simulink model "HPGR_2"  (Simulink 7.5)
settings: Solver=ode45  StartTime=0.0  StopTime=10.0  RelTol=1e-3
values from neighbouring files (symbols this model uses):
  n = 13    [CHANCADO_HPGR.m]    (also in Eficiencia_harnero_flujos.m; Granulometria10a.m; HARNERO_bajo_Tamano.m; Prechancado.m)
  X = [37.649701194 26.5631323454 18.9314553059 13.3865604245 9.46572765296 6.69328021227 3.95979797464 1.67332005307 0.707106781187 0.39686269666 0.25099800796 0.158113883008 ... (13 elements, 1x13)]    [matlab.mat]
  Xc = (s0 + D*(1-cos(alfaIP*pi/180)))*1000    [Capacidad_tratamiento_consumo_energia_especifica.m]    (also in Prechancado.m = 27.6127; programacion.m = x(1))
undefined symbols (not defined in the file or in its folder): alfa, faHPGR
settings Model: Creator=Lucho  LastModifiedBy=Lucho

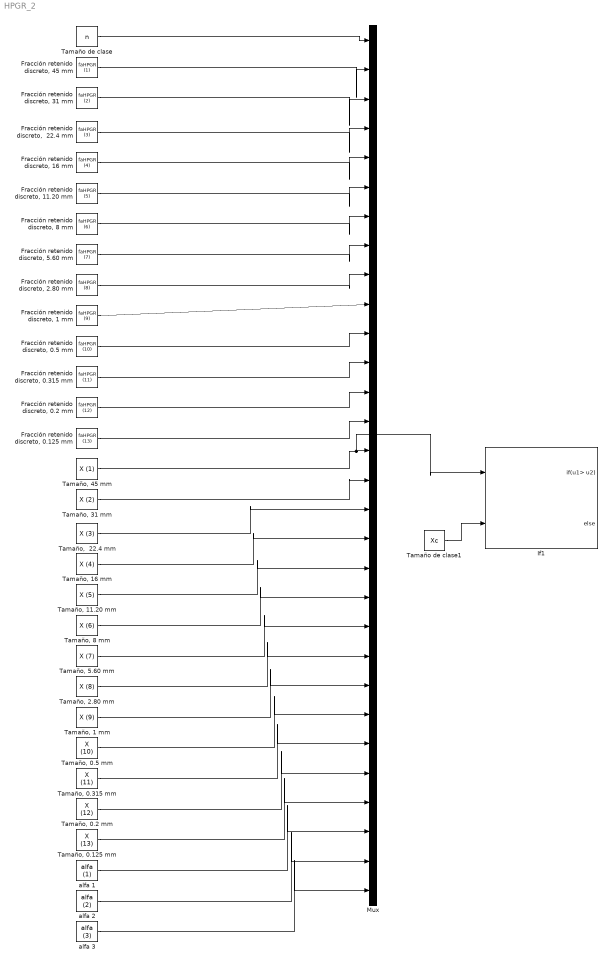
== system HPGR_2 ==
  "Fracción retenido discreto,  22.4 mm" : Constant  Value=faHPGR (3)  OutDataType=fixdt(1, 16)  OutScaling=2^0
  "Fracción retenido discreto, 0.125 mm" : Constant  Value=faHPGR (13)  OutDataType=fixdt(1, 16)  OutScaling=2^0
  "Fracción retenido discreto, 0.2 mm" : Constant  Value=faHPGR (12)  OutDataType=fixdt(1, 16)  OutScaling=2^0
  "Fracción retenido discreto, 0.315 mm" : Constant  Value=faHPGR (11)  OutDataType=fixdt(1, 16)  OutScaling=2^0
  "Fracción retenido discreto, 0.5 mm" : Constant  Value=faHPGR (10)  OutDataType=fixdt(1, 16)  OutScaling=2^0
  "Fracción retenido discreto, 1 mm" : Constant  Value=faHPGR (9)  OutDataType=fixdt(1, 16)  OutScaling=2^0
  "Fracción retenido discreto, 11.20 mm" : Constant  Value=faHPGR (5)  OutDataType=fixdt(1, 16)  OutScaling=2^0
  "Fracción retenido discreto, 16 mm" : Constant  Value=faHPGR (4)  OutDataType=fixdt(1, 16)  OutScaling=2^0
  "Fracción retenido discreto, 2.80 mm" : Constant  Value=faHPGR (8)  OutDataType=fixdt(1, 16)  OutScaling=2^0
  "Fracción retenido discreto, 31 mm" : Constant  Value=faHPGR (2)  OutDataType=fixdt(1, 16)  OutScaling=2^0
  "Fracción retenido discreto, 45 mm" : Constant  Value=faHPGR (1)  OutDataType=fixdt(1, 16)  OutScaling=2^0
  "Fracción retenido discreto, 5.60 mm" : Constant  Value=faHPGR (7)  OutDataType=fixdt(1, 16)  OutScaling=2^0
  "Fracción retenido discreto, 8 mm" : Constant  Value=faHPGR (6)  OutDataType=fixdt(1, 16)  OutScaling=2^0
  If1 : If  NumInputs=2  IfExpression=u1> u2
  Mux : Mux  Inputs=30
  Tamaño de clase : Constant  Value=n  OutDataType=fixdt(1, 16)  OutScaling=2^0
  Tamaño de clase1 : Constant  Value=Xc  OutDataType=fixdt(1, 16)  OutScaling=2^0
  "Tamaño,  22.4 mm" : Constant  Value=X (3)  OutDataType=fixdt(1, 16)  OutScaling=2^0
  "Tamaño, 0.125 mm" : Constant  Value=X (13)  OutDataType=fixdt(1, 16)  OutScaling=2^0
  "Tamaño, 0.2 mm" : Constant  Value=X (12)  OutDataType=fixdt(1, 16)  OutScaling=2^0
  "Tamaño, 0.315 mm" : Constant  Value=X (11)  OutDataType=fixdt(1, 16)  OutScaling=2^0
  "Tamaño, 0.5 mm" : Constant  Value=X (10)  OutDataType=fixdt(1, 16)  OutScaling=2^0
  "Tamaño, 1 mm" : Constant  Value=X (9)  OutDataType=fixdt(1, 16)  OutScaling=2^0
  "Tamaño, 11.20 mm" : Constant  Value=X (5)  OutDataType=fixdt(1, 16)  OutScaling=2^0
  "Tamaño, 16 mm" : Constant  Value=X (4)  OutDataType=fixdt(1, 16)  OutScaling=2^0
  "Tamaño, 2.80 mm" : Constant  Value=X (8)  OutDataType=fixdt(1, 16)  OutScaling=2^0
  "Tamaño, 31 mm" : Constant  Value=X (2)  OutDataType=fixdt(1, 16)  OutScaling=2^0
  "Tamaño, 45 mm" : Constant  Value=X (1)  OutDataType=fixdt(1, 16)  OutScaling=2^0
  "Tamaño, 5.60 mm" : Constant  Value=X (7)  OutDataType=fixdt(1, 16)  OutScaling=2^0
  "Tamaño, 8 mm" : Constant  Value=X (6)  OutDataType=fixdt(1, 16)  OutScaling=2^0
  alfa 1 : Constant  Value=alfa (1)  OutDataType=fixdt(1, 16)  OutScaling=2^0
  alfa 2 : Constant  Value=alfa (2)  OutDataType=fixdt(1, 16)  OutScaling=2^0
  alfa 3 : Constant  Value=alfa (3)  OutDataType=fixdt(1, 16)  OutScaling=2^0
  wires:
  Tamaño de clase/1 -> Mux/1
  "Fracción retenido discreto, 45 mm"/1 -> Mux/2
  "Fracción retenido discreto, 31 mm"/1 -> Mux/3
  "Fracción retenido discreto,  22.4 mm"/1 -> Mux/4
  "Fracción retenido discreto, 16 mm"/1 -> Mux/5
  "Fracción retenido discreto, 11.20 mm"/1 -> Mux/6
  "Fracción retenido discreto, 1 mm"/1 -> Mux/10
  "Fracción retenido discreto, 0.5 mm"/1 -> Mux/11
  "Fracción retenido discreto, 0.2 mm"/1 -> Mux/13
  "Fracción retenido discreto, 0.125 mm"/1 -> Mux/14
  "Fracción retenido discreto, 0.315 mm"/1 -> Mux/12
  "Tamaño, 45 mm"/1 -> Mux/15, If1/1
  "Tamaño, 31 mm"/1 -> Mux/16
  "Tamaño,  22.4 mm"/1 -> Mux/17
  "Tamaño, 16 mm"/1 -> Mux/18
  "Tamaño, 11.20 mm"/1 -> Mux/19
  "Tamaño, 8 mm"/1 -> Mux/20
  "Tamaño, 5.60 mm"/1 -> Mux/21
  "Tamaño, 2.80 mm"/1 -> Mux/22
  "Tamaño, 1 mm"/1 -> Mux/23
  "Tamaño, 0.5 mm"/1 -> Mux/24
  "Tamaño, 0.315 mm"/1 -> Mux/25
  "Tamaño, 0.2 mm"/1 -> Mux/26
  "Tamaño, 0.125 mm"/1 -> Mux/27
  alfa 1/1 -> Mux/28
  alfa 2/1 -> Mux/29
  alfa 3/1 -> Mux/30
  "Fracción retenido discreto, 8 mm"/1 -> Mux/7
  "Fracción retenido discreto, 5.60 mm"/1 -> Mux/8
  "Fracción retenido discreto, 2.80 mm"/1 -> Mux/9
  Tamaño de clase1/1 -> If1/2
